simulink model "SignalTestingModel_v1"  (R2021a)
settings: Solver=VariableStepAuto  StartTime=0.0  StopTime=10.0  RelTol=1e-3
settings Model: Creator=20204920  LastModifiedBy=20204920

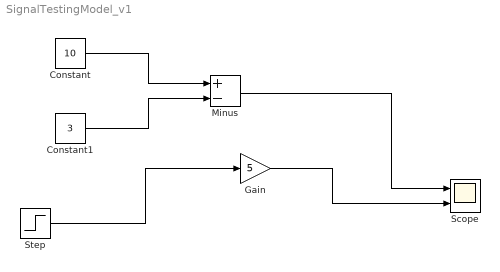
== system SignalTestingModel_v1 ==
  Constant : Constant  Value=10  OutDataTypeStr=int64
  Constant1 : Constant  Value=3  OutDataTypeStr=uint16
  Gain : Gain  Gain=5  OutDataTypeStr=double
  Minus : Sum  Inputs=+-
  Scope : Scope  NumInputPorts=2
  Step : Step  OutDataTypeStr=single  SampleTime=0
  wires:
  Constant/1 -> Minus/1
  Constant1/1 -> Minus/2
  Minus/1 -> Scope/1
  Step/1 -> Gain/1
  Gain/1 -> Scope/2
